simulink model "model1"  (R2024b)
settings: Solver=VariableStepAuto  StartTime=0.0  StopTime=20  RelTol=1e-3
settings Model: Creator=mehmetcanevi  LastModifiedBy=mehmetcanevi

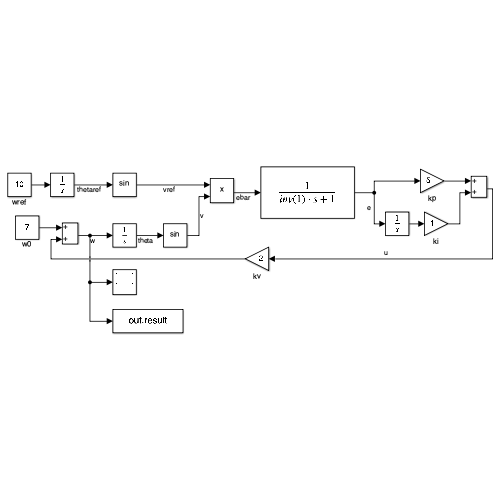
[thumbnail: Simulink's stored preview of the top-level diagram]
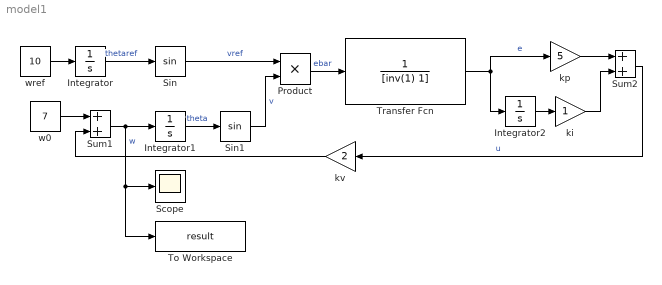
== system model1 ==
  Integrator : Integrator
  Integrator1 : Integrator
  Integrator2 : Integrator
  Product : Product
  Scope : Scope
  Sin : Trigonometry
  Sin1 : Trigonometry
  Sum1 : Sum
  Sum2 : Sum
  To Workspace : ToWorkspace  VariableName=result  SampleTime=-1
  Transfer Fcn : TransferFcn  Denominator=[inv(1) 1]
  ki : Gain
  kp : Gain  Gain=5
  kv : Gain  Gain=2
  w0 : Constant  Value=7
  wref : Constant  Value=10
  wires:
  Sin/1 -> Product/1  "vref"
  Sum2/1 -> kv/1  "u"
  Transfer Fcn/1 -> kp/1, Integrator2/1  "e"
  Integrator/1 -> Sin/1  "thetaref"
  Integrator2/1 -> ki/1
  kv/1 -> Sum1/2
  kp/1 -> Sum2/1
  Integrator1/1 -> Sin1/1  "theta"
  ki/1 -> Sum2/2
  wref/1 -> Integrator/1
  w0/1 -> Sum1/1
  Product/1 -> Transfer Fcn/1  "ebar"
  Sum1/1 -> Integrator1/1, To Workspace/1, Scope/1  "w"
  Sin1/1 -> Product/2  "v"
